simulink model "pid_series_sim"  (R2023a)
settings: Solver=VariableStepAuto  StartTime=0.0  StopTime=0.2  MaxStep=Ts  RelTol=1e-3
values from neighbouring files (symbols this model uses):
  g_awr = 1.6    [pid_ini_parallel.m]    (also in pid_ini_series.m = 1)
  Ki = Ki_s    (= 2356.19449019)    [pid_ini_parallel.m]    (also in pid_ini_series.m)
  Kp = (Ki_s*fp_s - Ki_s*fz_s + 2*pi*Kp_s*fp_s*fz_s)/(2*fp_s*fz_s*pi)    (= 42.5)    [pid_ini_parallel.m]    (also in pid_ini_series.m = 25)
  Ts = 50e-6    (= 5e-05)    [pid_ini_parallel.m]    (also in pid_ini_series.m)
  u_max = 5.5    [pid_ini_parallel.m]    (also in pid_ini_series.m)
  u_min = -u_max    (= -5.5)    [pid_ini_parallel.m]    (also in pid_ini_series.m)
libraries: cstblocks x8
settings Model: Creator=Michael Peter  LastModifiedBy=Michael Peter

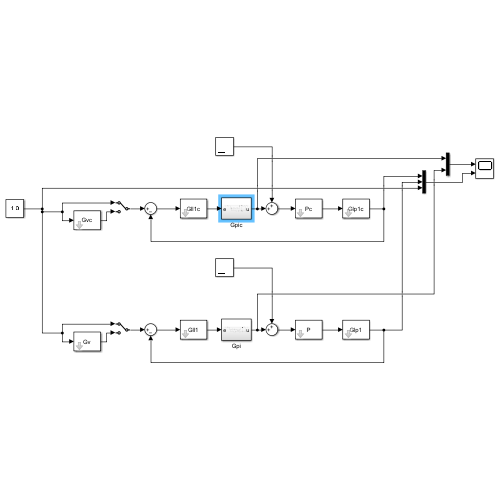
[thumbnail: Simulink's stored preview of the top-level diagram]
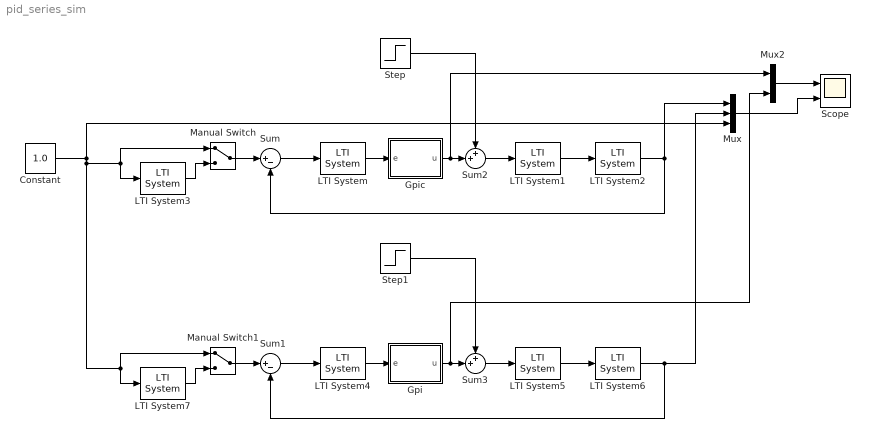
== system pid_series_sim ==
  Constant : Constant  Value=1.0
  Gpi : Subsystem
  Gpic : Subsystem
  LTI System : cstblocks/LTI System  sys=Gll1c  IC=[]
  LTI System1 : cstblocks/LTI System  sys=Pc  IC=[]
  LTI System2 : cstblocks/LTI System  sys=Glp1c  IC=[]
  LTI System3 : cstblocks/LTI System  sys=Gvc  IC=[]
  LTI System4 : cstblocks/LTI System  sys=Gll1  IC=[]
  LTI System5 : cstblocks/LTI System  sys=P  IC=[]
  LTI System6 : cstblocks/LTI System  sys=Glp1  IC=[]
  LTI System7 : cstblocks/LTI System  sys=Gv  IC=[]
  Manual Switch : ManualSwitch
  Manual Switch1 : ManualSwitch
  Mux : Mux  Inputs=3
  Mux2 : Mux  Inputs=2
  Scope : Scope  NumInputPorts=2
  Step : Step  Time=0.12  After=3.5  SampleTime=0
  Step1 : Step  Time=0.12  After=3.5  SampleTime=0
  Sum : Sum  Inputs=|+-
  Sum1 : Sum  Inputs=|+-
  Sum2 : Sum  Inputs=++|
  Sum3 : Sum  Inputs=++|
  wires:
  LTI System1/1 -> LTI System2/1
  LTI System/1 -> Gpic/1(e)
  Sum/1 -> LTI System/1
  LTI System2/1 -> Mux/1, Sum/2
  Gpic/1(u) -> Mux2/1, Sum2/2
  Sum2/1 -> LTI System1/1
  Mux/1 -> Scope/2
  Step/1 -> Sum2/1
  Manual Switch/1 -> Sum/1
  LTI System3/1 -> Manual Switch/2
  LTI System7/1 -> Manual Switch1/2
  Manual Switch1/1 -> Sum1/1
  Step1/1 -> Sum3/1
  Constant/1 -> LTI System7/1, Manual Switch1/1, Manual Switch/1, LTI System3/1, Mux/3
  Sum3/1 -> LTI System5/1
  Gpi/1(u) -> Mux2/2, Sum3/2
  LTI System6/1 -> Mux/2, Sum1/2
  Sum1/1 -> LTI System4/1
  LTI System4/1 -> Gpi/1(e)
  LTI System5/1 -> LTI System6/1
  Mux2/1 -> Scope/1

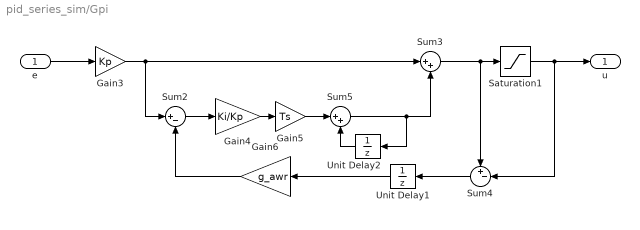
== system pid_series_sim/Gpi ==
  e : Inport
  Gain3 : Gain  Gain=Kp
  Gain4 : Gain  Gain=Ki/Kp
  Gain5 : Gain  Gain=Ts
  Gain6 : Gain  Gain=g_awr
  Saturation1 : Saturate  UpperLimit=u_max  LowerLimit=u_min
  Sum2 : Sum  Inputs=|+-
  Sum3 : Sum  Inputs=|++
  Sum4 : Sum  Inputs=+-|
  Sum5 : Sum  Inputs=|++
  Unit Delay1 : UnitDelay  SampleTime=Ts  HasFrameUpgradeWarning=on
  Unit Delay2 : UnitDelay  SampleTime=Ts  HasFrameUpgradeWarning=on
  u : Outport
  wires:
  Gain6/1 -> Sum2/2
  e/1 -> Gain3/1
  Sum5/1 -> Unit Delay2/1, Sum3/2
  Gain5/1 -> Sum5/1
  Gain3/1 -> Sum3/1, Sum2/1
  Sum2/1 -> Gain4/1
  Gain4/1 -> Gain5/1
  Sum4/1 -> Unit Delay1/1
  Sum3/1 -> Sum4/1, Saturation1/1
  Saturation1/1 -> u/1, Sum4/2
  Unit Delay1/1 -> Gain6/1
  Unit Delay2/1 -> Sum5/2

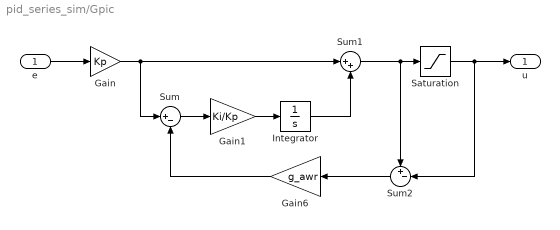
== system pid_series_sim/Gpic ==
  e : Inport
  Gain : Gain  Gain=Kp
  Gain1 : Gain  Gain=Ki/Kp
  Gain6 : Gain  Gain=g_awr
  Integrator : Integrator
  Saturation : Saturate  UpperLimit=u_max  LowerLimit=u_min
  Sum : Sum  Inputs=|+-
  Sum1 : Sum  Inputs=|++
  Sum2 : Sum  Inputs=+-|
  u : Outport
  wires:
  Saturation/1 -> u/1, Sum2/2
  Sum1/1 -> Sum2/1, Saturation/1
  Integrator/1 -> Sum1/2
  Gain1/1 -> Integrator/1
  Sum2/1 -> Gain6/1
  Gain/1 -> Sum1/1, Sum/1
  Sum/1 -> Gain1/1
  e/1 -> Gain/1
  Gain6/1 -> Sum/2
